simulink library "LossModelib"  (Simulink 7.8)
settings: Solver=ode45  StartTime=0.0  StopTime=10.0  RelTol=1e-3
undefined symbols (not defined in the file or in its folder): Esw_Erec, Esw_Off, Esw_On, LossSpec_Diode, LossSpec_IGBT, Page_Temp_C
libraries: simulink x12, powerlib_extras x9, fl_lib x8, powerlib x4, nesl_utility x4
settings Model: Creator=at4494  LastModifiedBy=at4494

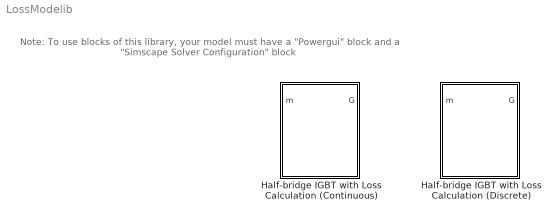
== system LossModelib ==
  note: Note: To use blocks of this library,  your model must have a "Powergui" block
      | and a "Simscape Solver Configuration" block
  Half-bridge IGBT with Loss Calculation (Continuous) : Subsystem  mask(Half-Bridge IGBT with thermal model and losses calculation){Ron=1e-3, IGBT_Type=Fuji: Half-bridge IGBT 600V/150A, PlotSpec_IGBT_On=off, ShowDataSheet_IGBT_On=off, Diode_Type=Fuji: Half-bridge IGBT 600V/150A, PlotSpec_Diode_On=off, ShowDataSheet_Diode_On=off, Tj_Init=40, PulseDuration=1e-6}
      mask prompts: Ron "Internal resistance Ron (Ohms):"; IGBT_Type "IGBT Type:"; PlotSpec_IGBT_On "Plot IGBT Characteristics"; ShowDataSheet_IGBT_On "Show Data Sheet"; Diode_Type "Diode Type:"; PlotSpec_Diode_On "Plot Diode Characteristics"; ShowDataSheet_Diode_On "Show Data Sheet"; Tj_Init "Initial Junction Temperature (degrees Celsius):"; PulseDuration "Pulse Duration for Energy-to-Power conversion (s):"
      mask init:
      | %
      | BlockName=gcb;
      | Rs=1e6;
      | Cs=inf;
      | %Tj0=273+ Tj_Init;
      | Tj0=Tj_Init;
      | %
      | load LossSpec_IGBT_Library
      | n=IGBT_Type;
      | % Add a row with 0 values for Eon and Eoff
      | E0_On=zeros(1,length(LossSpec_IGBT(n).Eon));
      | Esw_On(:,:,1)=[E0_On;LossSpec_IGBT(n).Eon(1,:)];
      | Esw_On(:,:,2)=[E0_On;LossSpec_IGBT(n).Eon(2,:)];
      | E0_Off=zeros(1,length(LossSpec_IGBT(n).Eoff));
      | Esw_Off(:,:,1)=[E0_Off;LossSpec_IGBT(n).Eoff(1,:)];
      | Esw_Off(:,:,2)=[E0_Off;LossSpec_IGBT(n).Eoff(2,:)];
      | % Create a two-element vector for Vcc (first value = 0)
      | Vcc_Esw_On=[0 LossSpec_IGBT(n).Vcc_Eon];
      | Vcc_Esw_Off=[0 LossSpec_IGBT(n).Vcc_Eoff];
      | if PlotSpec_IGBT_On==1
      |     PlotSpec1_IGBT(LossSpec_IGBT(n))
      |     set_param(BlockName,'PlotSpec_IGBT_On', 'off')
      | end
      | %
      | load LossSpec_Diode_Library
      | m=Diode_Type;
      | % Add a row with 0 values for Erec
      | E0_Erec=zeros(1,length(LossSpec_Diode(m).Erec));
      | Esw_Erec(:,:,1)=[E0_Erec;LossSpec_Diode(m).Erec(1,:)];
      | Esw_Erec(:,:,2)=[E0_Erec;LossSpec_Diode(m).Erec(2,:)];
      | % Create a two-element vector for Vcc (first value = 0)
      | Vcc_Esw_Erec=[0 LossSpec_Diode(m).Vcc_Erec];
      | if PlotSpec_Diode_On==1
      |     PlotSpec1_Diode(LossSpec_Diode(m))
      |     set_param(BlockName,'PlotSpec_Diode_On', 'off')
      | end
      | if ShowDataSheet_IGBT_On==1
      |     switch n
      |         case 1
      |     open('Spec_Fuji_IGBT600V150A.pdf')
      |         case 2
      |     open('Spec_ABB_IGBT1700V800A.pdf')
      |         case 3
      |     open('Spec_ABB_IGBT3300V250A.pdf')
      |     end
      |     set_param(BlockName,'ShowDataSheet_IGBT_On', 'off')
      | end
      | if ShowDataSheet_Diode_On==1
      |     switch m
      |         case 1
      |     open('Spec_Fuji_IGBT600V150A.pdf')
      |         case 2
      |     open('Spec_ABB_IGBT1700V800A.pdf')
      |         case 3
      |     open('Spec_ABB_IGBT3300V250A.pdf')
      |     end
      |     set_param(BlockName,'ShowDataSheet_Diode_On', 'off')
      | end
      mask StyleString: edit,popup(Fuji: Half-bridge IGBT 600V/150A|ABB: IGBT Chopper 1700V/800A|ABB: Half-Bridge IGBT 3300V/250A),checkbox,checkbox,popup(Fuji: Half-bridge IGBT 600V/150A|ABB: IGBT Chopper 1700V/800A|ABB: Half-Bridge IGBT 3300V/250A),checkbox,checkbox,edit,edit
      mask Display:
      | dX=0.02;
      | dY=0.05;
      | plot([0.19 0.292 0.292]+dX,[0.575 0.575 0.685]+dY)
      | plot([0.19 0.292 0.292]+dX,[0.195 0.195 0.305]+dY)
      | plot([0.476 0.794]+dX,[0.455 0.455]+dY)
      | plot([0.476 0.476 0.346 0.346 0.346 0.346 0.476 0.476]+dX,[0.850 0.732 0.680 0.723 0.546 0.622 0.575 0.455 ]+dY)
      | patch([0.476 0.427 0.415 0.476]+dX,[0.576 0.610 0.576 0.576]+dY)
      | %
      | plot([0.476 0.476 0.346 0.346 0.346 0.346 0.476 0.476]+dX,[0.850 0.732 0.680 0.723 0.546 0.622 0.575 0.455 ]-0.385+dY)
      | patch([0.476 0.427 0.415 0.476]+dX,[0.576 0.610 0.576 0.576]-0.385+dY)
      | %
      | plot([0.614 0.614 0.476]+dX,[0.776 0.507 0.507]+dY)
      | plot([0.614 0.476]+dX,[0.776 0.776]+dY)
      | plot([0.577 0.650]+dX,[0.679 0.679]+dY)
      | patch([0.577 0.650  0.614 0.577]+dX,[0.619 0.619 0.679 0.619]+dY)
      | %
      | plot([0.614 0.614 0.476]+dX,[0.776 0.507 0.507]-0.385+dY)
      | plot([0.614 0.476]+dX,[0.776 0.776]-0.385+dY)
      | plot([0.577 0.650]+dX,[0.679 0.679]-0.385+dY)
      | patch([0.577 0.650  0.614 0.577]+dX,[0.619 0.619 0.679 0.619]-0.385+dY)
      | %
      | port_label('RConn', 1,'+');
      | port_label('RConn', 2,'-');
      | port_label('LConn', 1,'A');
      | color('red');
      | port_label('LConn', 2,'H');
      | color('blue');
      | port_label('input', 1,'G');
  Half-bridge IGBT with Loss Calculation (Discrete) : Subsystem  mask(Half-Bridge IGBT with thermal model & losses calculation){Ron=1e-3, IGBT_Type=Fuji: Half-bridge IGBT 600V/150A, PlotSpec_IGBT_On=off, ShowDataSheet_IGBT_On=off, Diode_Type=Fuji: Half-bridge IGBT 600V/150A, PlotSpec_Diode_On=off, ShowDataSheet_Diode_On=off, Tj_Init=40, PulseDuration=1e-6, Ts=1e-6}
      mask prompts: Ron "Internal resistance Ron (Ohms):"; IGBT_Type "IGBT Type:"; PlotSpec_IGBT_On "Plot IGBT Characteristics"; ShowDataSheet_IGBT_On "Show Data Sheet"; Diode_Type "Diode Type:"; PlotSpec_Diode_On "Plot Diode Characteristics"; ShowDataSheet_Diode_On "Show Data Sheet"; Tj_Init "Initial Junction Temperature (degrees Celsius):"; PulseDuration "Pulse Duration for Energy-to-Power conversion (s):"; Ts "Sample time (s):"
      mask init:
      | %
      | BlockName=gcb;
      | Rs=1e6;
      | Cs=inf;
      | %Tj0=273+ Tj_Init;
      | Tj0=Tj_Init;
      | %
      | load LossSpec_IGBT_Library
      | n=IGBT_Type;
      | % Add a row with 0 values for Eon and Eoff
      | E0_On=zeros(1,length(LossSpec_IGBT(n).Eon));
      | Esw_On(:,:,1)=[E0_On;LossSpec_IGBT(n).Eon(1,:)];
      | Esw_On(:,:,2)=[E0_On;LossSpec_IGBT(n).Eon(2,:)];
      | E0_Off=zeros(1,length(LossSpec_IGBT(n).Eoff));
      | Esw_Off(:,:,1)=[E0_Off;LossSpec_IGBT(n).Eoff(1,:)];
      | Esw_Off(:,:,2)=[E0_Off;LossSpec_IGBT(n).Eoff(2,:)];
      | % Create a two-element vector for Vcc (first value = 0)
      | Vcc_Esw_On=[0 LossSpec_IGBT(n).Vcc_Eon];
      | Vcc_Esw_Off=[0 LossSpec_IGBT(n).Vcc_Eoff];
      | if PlotSpec_IGBT_On==1
      |     PlotSpec1_IGBT(LossSpec_IGBT(n))
      |     set_param(BlockName,'PlotSpec_IGBT_On', 'off')
      | end
      | %
      | load LossSpec_Diode_Library
      | m=Diode_Type;
      | % Add a row with 0 values for Erec
      | E0_Erec=zeros(1,length(LossSpec_Diode(m).Erec));
      | Esw_Erec(:,:,1)=[E0_Erec;LossSpec_Diode(m).Erec(1,:)];
      | Esw_Erec(:,:,2)=[E0_Erec;LossSpec_Diode(m).Erec(2,:)];
      | % Create a two-element vector for Vcc (first value = 0)
      | Vcc_Esw_Erec=[0 LossSpec_Diode(m).Vcc_Erec];
      | if PlotSpec_Diode_On==1
      |     PlotSpec1_Diode(LossSpec_Diode(m))
      |     set_param(BlockName,'PlotSpec_Diode_On', 'off')
      | end
      | if ShowDataSheet_IGBT_On==1
      |     switch n
      |         case 1
      |     open('Fuji_IGBT600V150A.pdf')
      |         case 2
      |     open('ABB_IGBT1700V800A.pdf')
      |         case 3
      |     open('ABB_IGBT3300V250A.pdf')
      |     end
      |     set_param(BlockName,'ShowDataSheet_IGBT_On', 'off')
      | end
      | if ShowDataSheet_Diode_On==1
      |     switch m
      |         case 1
      |     open('Fuji_IGBT600V150A.pdf')
      |         case 2
      |     open('ABB_IGBT1700V800A.pdf')
      |         case 3
      |     open('ABB_IGBT3300V250A.pdf')
      |     end
      |     set_param(BlockName,'ShowDataSheet_Diode_On', 'off')
      | end
      mask StyleString: edit,popup(Fuji: Half-bridge IGBT 600V/150A|ABB: IGBT Chopper 1700V/800A|ABB: Half-Bridge IGBT 3300V/250A),checkbox,checkbox,popup(Fuji: Half-bridge IGBT 600V/150A|ABB: IGBT Chopper 1700V/800A|ABB: Half-Bridge IGBT 3300V/250A),checkbox,checkbox,edit,edit,edit
      mask Display:
      | dX=0.02;
      | dY=0.05;
      | plot([0.19 0.292 0.292]+dX,[0.575 0.575 0.685]+dY)
      | plot([0.19 0.292 0.292]+dX,[0.195 0.195 0.305]+dY)
      | plot([0.476 0.794]+dX,[0.455 0.455]+dY)
      | plot([0.476 0.476 0.346 0.346 0.346 0.346 0.476 0.476]+dX,[0.850 0.732 0.680 0.723 0.546 0.622 0.575 0.455 ]+dY)
      | patch([0.476 0.427 0.415 0.476]+dX,[0.576 0.610 0.576 0.576]+dY)
      | %
      | plot([0.476 0.476 0.346 0.346 0.346 0.346 0.476 0.476]+dX,[0.850 0.732 0.680 0.723 0.546 0.622 0.575 0.455 ]-0.385+dY)
      | patch([0.476 0.427 0.415 0.476]+dX,[0.576 0.610 0.576 0.576]-0.385+dY)
      | %
      | plot([0.614 0.614 0.476]+dX,[0.776 0.507 0.507]+dY)
      | plot([0.614 0.476]+dX,[0.776 0.776]+dY)
      | plot([0.577 0.650]+dX,[0.679 0.679]+dY)
      | patch([0.577 0.650  0.614 0.577]+dX,[0.619 0.619 0.679 0.619]+dY)
      | %
      | plot([0.614 0.614 0.476]+dX,[0.776 0.507 0.507]-0.385+dY)
      | plot([0.614 0.476]+dX,[0.776 0.776]-0.385+dY)
      | plot([0.577 0.650]+dX,[0.679 0.679]-0.385+dY)
      | patch([0.577 0.650  0.614 0.577]+dX,[0.619 0.619 0.679 0.619]-0.385+dY)
      | %
      | port_label('RConn', 1,'+');
      | port_label('RConn', 2,'-');
      | port_label('LConn', 1,'A');
      | color('red');
      | port_label('LConn', 2,'H');
      | color('blue');
      | port_label('input', 1,'G');

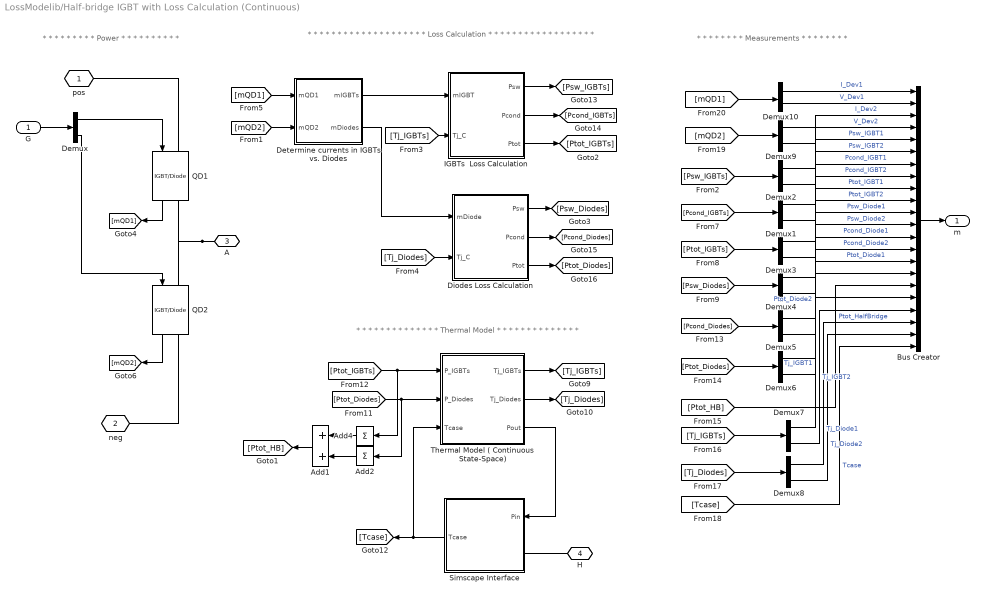
== system LossModelib/Half-bridge IGBT with Loss Calculation (Continuous) ==
  note: * * * * * * * * * Power * * * * * * * * * *
  note: * * * * * * * * * * * * * * * * * * * * Loss Calculation * * * * * * * * * * * * * * * * * *
  note: * * * * * * * * * * * * * * Thermal Model * * * * * * * * * * * * * *
  note: * * * * * * * * Measurements * * * * * * * *
  G : Inport  PortDimensions=2
  Add1 : Sum
  Add2 : Sum  Inputs=+
  Add4 : Sum  Inputs=+
  Bus Creator : BusCreator  Inputs=22
  Demux{,1..10} (11 alike) : Demux  Outputs=2
  Determine currents in IGBTs vs. Diodes : Subsystem
  Diodes Loss Calculation : Subsystem
  IGBTs  Loss Calculation : Subsystem
  QD1 : powerlib/Power Electronics/IGBT//Diode  Ron=Ron  Rs=Rs  Cs=Cs  Measurements=on
  QD2 : powerlib/Power Electronics/IGBT//Diode  Ron=Ron  Rs=Rs  Cs=Cs  Measurements=on
  Simscape Interface : Subsystem
  Thermal Model ( Continuous State-Space) : Subsystem  mask(State-Space Thermal Model (Junction-to-Case)){Zth_IGBT=[ LossSpec_IGBT(n).Rth_jc    LossSpec_IGBT(n).Cth_j ], Zth_Diode=[ LossSpec_Diode(m).Rth_jc    LossSpec_Diode(m).Cth_j ], Tj0=Tj0}
      mask prompts: Zth_IGBT "IGBT Thermal Impedance [ Rth (K/W)  Cth (J/K) ]:"; Zth_Diode "Diode Thermal Impedance [ Rth (K/W)  Cth (J/K) ]:"; Tj0 "Junction Initial Temperature (C)"
      mask init:
      | %
      | Rth_IGBT= Zth_IGBT(1);
      | Cth_IGBT= Zth_IGBT(2);
      | Rth_Diode= Zth_Diode(1);
      | Cth_Diode= Zth_Diode(2);
      | %
      | Ac_IGBT= -1/(Rth_IGBT*Cth_IGBT);
      | Bc_IGBT= [ 1/(Rth_IGBT*Cth_IGBT)  1/Cth_IGBT ];
      | Cc_IGBT= [ 1; 1/Rth_IGBT ];
      | Dc_IGBT= [ 0  0; -1/Rth_IGBT 0 ];
      | %
      | Ac_Diode= -1/(Rth_Diode*Cth_Diode);
      | Bc_Diode= [ 1/(Rth_Diode*Cth_Diode)  1/Cth_Diode ];
      | Cc_Diode= [ 1; 1/Rth_Diode ];
      | Dc_Diode= [ 0  0; -1/Rth_Diode 0 ];
      | %
      | x0c=Tj0;
      | %
  pos : PMIOPort  Port=1  Side=Right
  neg : PMIOPort  Port=2  Side=Right
  A : PMIOPort  Port=3  Side=Left
  H : PMIOPort  Port=4  Side=Left
  m : Outport
  wires:
  Simscape Interface/1(Tcase) -> Thermal Model ( Continuous State-Space)/3(Tcase), [Tcase]
  Thermal Model ( Continuous State-Space)/3(Pout) -> Simscape Interface/1(Pin)
  [Ptot_IGBTs] -> Thermal Model ( Continuous State-Space)/1(P_IGBTs), Add4/1
  [Ptot_Diodes] -> Thermal Model ( Continuous State-Space)/2(P_Diodes), Add2/1
  Thermal Model ( Continuous State-Space)/1(Tj_IGBTs) -> [Tj_IGBTs]
  Thermal Model ( Continuous State-Space)/2(Tj_Diodes) -> [Tj_Diodes]
  QD1/1 -> [mQD1]
  QD2/1 -> [mQD2]
  Demux/1 -> QD1/1
  G/1 -> Demux/1
  Demux/2 -> QD2/1
  IGBTs  Loss Calculation/2(Pcond) -> [Pcond_IGBTs]
  [mQD1] -> Determine currents in IGBTs vs. Diodes/1(mQD1)
  [mQD2] -> Determine currents in IGBTs vs. Diodes/2(mQD2)
  Determine currents in IGBTs vs. Diodes/1(mIGBTs) -> IGBTs  Loss Calculation/1(mIGBT)
  Determine currents in IGBTs vs. Diodes/2(mDiodes) -> Diodes Loss Calculation/1(mDiode)
  IGBTs  Loss Calculation/1(Psw) -> [Psw_IGBTs]
  [Tj_IGBTs] -> IGBTs  Loss Calculation/2(Tj_C)
  [Tj_Diodes] -> Diodes Loss Calculation/2(Tj_C)
  IGBTs  Loss Calculation/3(Ptot) -> [Ptot_IGBTs]
  Diodes Loss Calculation/1(Psw) -> [Psw_Diodes]
  Diodes Loss Calculation/2(Pcond) -> [Pcond_Diodes]
  Diodes Loss Calculation/3(Ptot) -> [Ptot_Diodes]
  Bus Creator/1 -> m/1
  [Psw_IGBTs] -> Demux2/1
  [Pcond_IGBTs] -> Demux1/1
  [Ptot_IGBTs] -> Demux3/1
  [Psw_Diodes] -> Demux4/1
  [Pcond_Diodes] -> Demux5/1
  [Ptot_Diodes] -> Demux6/1
  Add1/1 -> [Ptot_HB]
  [Tj_IGBTs] -> Demux7/1
  [Tj_Diodes] -> Demux8/1
  [mQD1] -> Demux10/1
  [mQD2] -> Demux9/1
  Demux10/1 -> Bus Creator/1  "I_Dev1"
  Demux10/2 -> Bus Creator/2  "V_Dev1"
  Demux9/1 -> Bus Creator/3  "I_Dev2"
  Demux9/2 -> Bus Creator/4  "V_Dev2"
  Demux2/1 -> Bus Creator/5  "Psw_IGBT1"
  Demux2/2 -> Bus Creator/6  "Psw_IGBT2"
  Demux1/1 -> Bus Creator/7  "Pcond_IGBT1"
  Demux1/2 -> Bus Creator/8  "Pcond_IGBT2"
  Demux3/1 -> Bus Creator/9  "Ptot_IGBT1"
  Demux3/2 -> Bus Creator/10  "Ptot_IGBT2"
  Demux4/1 -> Bus Creator/11  "Psw_Diode1"
  Demux4/2 -> Bus Creator/12  "Psw_Diode2"
  Demux5/1 -> Bus Creator/13  "Pcond_Diode1"
  Demux5/2 -> Bus Creator/14  "Pcond_Diode2"
  Demux6/1 -> Bus Creator/15  "Ptot_Diode1"
  Demux6/2 -> Bus Creator/16  "Ptot_Diode2"
  [Ptot_HB] -> Bus Creator/17  "Ptot_HalfBridge"
  Demux7/1 -> Bus Creator/18  "Tj_IGBT1"
  Demux7/2 -> Bus Creator/19  "Tj_IGBT2"
  Demux8/1 -> Bus Creator/20  "Tj_Diode1"
  Demux8/2 -> Bus Creator/21  "Tj_Diode2"
  [Tcase] -> Bus Creator/22  "Tcase"
  Add4/1 -> Add1/1
  Add2/1 -> Add1/2
  connections:
  H/RConn1 -- Simscape Interface/LConn1
  A/RConn1 -- QD2/LConn1 -- QD1/RConn1
  pos/RConn1 -- QD1/LConn1
  neg/RConn1 -- QD2/RConn1

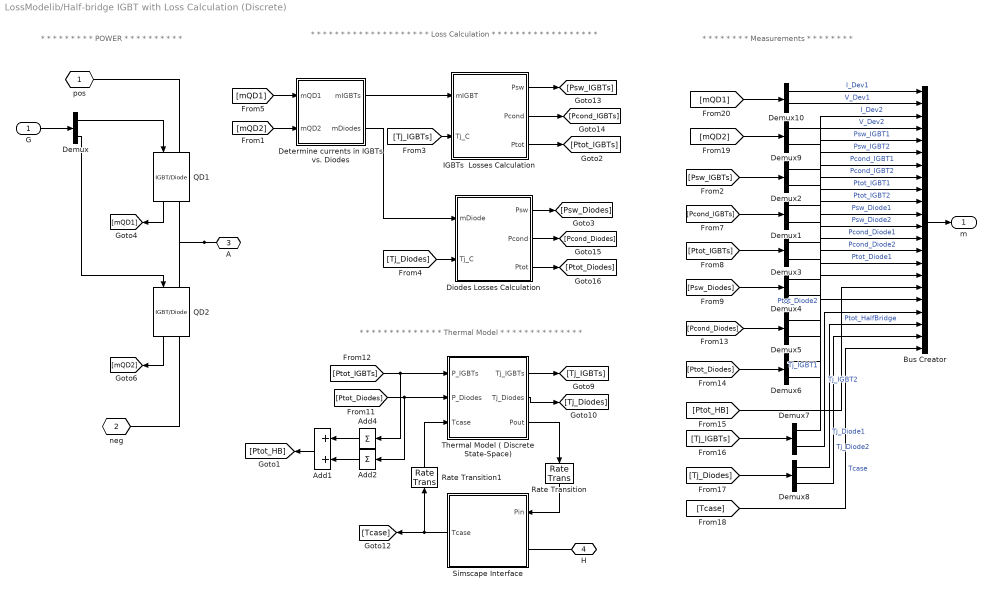
== system LossModelib/Half-bridge IGBT with Loss Calculation (Discrete) ==
  note: * * * * * * * * * POWER * * * * * * * * * *
  note: * * * * * * * * * * * * * * * * * * * * Loss Calculation * * * * * * * * * * * * * * * * * *
  note: * * * * * * * * * * * * * * Thermal Model * * * * * * * * * * * * * *
  note: * * * * * * * * Measurements * * * * * * * *
  G : Inport  PortDimensions=2
  Add1 : Sum
  Add2 : Sum  Inputs=+
  Add4 : Sum  Inputs=+
  Bus Creator : BusCreator  Inputs=22
  Demux{,1..10} (11 alike) : Demux  Outputs=2
  Determine currents in IGBTs vs. Diodes : Subsystem
  Diodes Losses Calculation : Subsystem
  IGBTs  Losses Calculation : Subsystem
  QD1 : powerlib/Power Electronics/IGBT//Diode  Ron=Ron  Rs=Rs  Cs=Cs  Measurements=on
  QD2 : powerlib/Power Electronics/IGBT//Diode  Ron=Ron  Rs=Rs  Cs=Cs  Measurements=on
  Rate Transition : RateTransition  OutPortSampleTime=100e-6
  Rate Transition1 : RateTransition  OutPortSampleTime=Ts
  Simscape Interface : Subsystem
  Thermal Model ( Discrete State-Space) : Subsystem  mask(State-Space Thermal Model (Junction-to-Case)){Zth_IGBT=[ LossSpec_IGBT(n).Rth_jc    LossSpec_IGBT(n).Cth_j ], Zth_Diode=[ LossSpec_Diode(m).Rth_jc    LossSpec_Diode(m).Cth_j], Tj0=Tj0, Ts=Ts}
      mask prompts: Zth_IGBT "IGBT Thermal Impedance [ Rth (K/W)  Cth (J/K) ]:"; Zth_Diode "Diode Thermal Impedance [ Rth (K/W)  Cth (J/K) ]:"; Tj0 "Junction Initial Temperature (C)"; Ts "Sample time (s):"
      mask init:
      | %
      | Rth_IGBT= Zth_IGBT(1);
      | Cth_IGBT= Zth_IGBT(2);
      | Rth_Diode= Zth_Diode(1);
      | Cth_Diode= Zth_Diode(2);
      | %
      | Ac_IGBT= -1/(Rth_IGBT*Cth_IGBT);
      | Bc_IGBT= [ 1/(Rth_IGBT*Cth_IGBT)  1/Cth_IGBT ];
      | Cc_IGBT= [ 1; 1/Rth_IGBT ];
      | Dc_IGBT= [ 0  0; -1/Rth_IGBT 0 ];
      | %
      | Ac_Diode= -1/(Rth_Diode*Cth_Diode);
      | Bc_Diode= [ 1/(Rth_Diode*Cth_Diode)  1/Cth_Diode ];
      | Cc_Diode= [ 1; 1/Rth_Diode ];
      | Dc_Diode= [ 0  0; -1/Rth_Diode 0 ];
      | %
      | x0c=Tj0;
      | %
      | %  Conversion to discrete transfer function
      | nstates = size(Ac_IGBT,1);
      | invexp = inv(eye(nstates) - (Ts/2)*Ac_IGBT);
      | Ad_IGBT = invexp*(eye(nstates) + (Ts/2)*Ac_IGBT);
      | Bd_IGBT = invexp*Bc_IGBT;
      | Cd_IGBT = Cc_IGBT*invexp*Ts;
      | Dd_IGBT = Cc_IGBT*invexp*Bc_IGBT*(Ts/2) + Dc_IGBT;
      | %
      | x0c=Tj0;
      | I=eye(size(Ac_IGBT));
      | x0d=(I-Ac_IGBT*Ts/2)*x0c/Ts;
      | %
      | %  Conversion to discrete transfer function
      | nstates = size(Ac_Diode,1);
      | invexp = inv(eye(nstates) - (Ts/2)*Ac_Diode);
      | Ad_Diode = invexp*(eye(nstates) + (Ts/2)*Ac_Diode);
      | Bd_Diode = invexp*Bc_Diode;
      | Cd_Diode = Cc_Diode*invexp*Ts;
      | Dd_Diode = Cc_Diode*invexp*Bc_Diode*(Ts/2) + Dc_Diode;
      | %
  pos : PMIOPort  Port=1  Side=Right
  neg : PMIOPort  Port=2  Side=Right
  A : PMIOPort  Port=3  Side=Left
  H : PMIOPort  Port=4  Side=Left
  m : Outport
  wires:
  Simscape Interface/1(Tcase) -> [Tcase], Rate Transition1/1
  Thermal Model ( Discrete State-Space)/3(Pout) -> Rate Transition/1
  [Ptot_IGBTs] -> Add4/1, Thermal Model ( Discrete State-Space)/1(P_IGBTs)
  [Ptot_Diodes] -> Add2/1, Thermal Model ( Discrete State-Space)/2(P_Diodes)
  Thermal Model ( Discrete State-Space)/1(Tj_IGBTs) -> [Tj_IGBTs]
  Thermal Model ( Discrete State-Space)/2(Tj_Diodes) -> [Tj_Diodes]
  QD1/1 -> [mQD1]
  QD2/1 -> [mQD2]
  Demux/1 -> QD1/1
  G/1 -> Demux/1
  Demux/2 -> QD2/1
  IGBTs  Losses Calculation/2(Pcond) -> [Pcond_IGBTs]
  [mQD1] -> Determine currents in IGBTs vs. Diodes/1(mQD1)
  [mQD2] -> Determine currents in IGBTs vs. Diodes/2(mQD2)
  Determine currents in IGBTs vs. Diodes/1(mIGBTs) -> IGBTs  Losses Calculation/1(mIGBT)
  Determine currents in IGBTs vs. Diodes/2(mDiodes) -> Diodes Losses Calculation/1(mDiode)
  IGBTs  Losses Calculation/1(Psw) -> [Psw_IGBTs]
  [Tj_IGBTs] -> IGBTs  Losses Calculation/2(Tj_C)
  [Tj_Diodes] -> Diodes Losses Calculation/2(Tj_C)
  IGBTs  Losses Calculation/3(Ptot) -> [Ptot_IGBTs]
  Diodes Losses Calculation/1(Psw) -> [Psw_Diodes]
  Diodes Losses Calculation/2(Pcond) -> [Pcond_Diodes]
  Diodes Losses Calculation/3(Ptot) -> [Ptot_Diodes]
  Bus Creator/1 -> m/1
  [Psw_IGBTs] -> Demux2/1
  [Pcond_IGBTs] -> Demux1/1
  [Ptot_IGBTs] -> Demux3/1
  [Psw_Diodes] -> Demux4/1
  [Pcond_Diodes] -> Demux5/1
  [Ptot_Diodes] -> Demux6/1
  Add1/1 -> [Ptot_HB]
  [Tj_IGBTs] -> Demux7/1
  [Tj_Diodes] -> Demux8/1
  [mQD1] -> Demux10/1
  [mQD2] -> Demux9/1
  Demux10/1 -> Bus Creator/1  "I_Dev1"
  Demux10/2 -> Bus Creator/2  "V_Dev1"
  Demux9/1 -> Bus Creator/3  "I_Dev2"
  Demux9/2 -> Bus Creator/4  "V_Dev2"
  Demux2/1 -> Bus Creator/5  "Psw_IGBT1"
  Demux2/2 -> Bus Creator/6  "Psw_IGBT2"
  Demux1/1 -> Bus Creator/7  "Pcond_IGBT1"
  Demux1/2 -> Bus Creator/8  "Pcond_IGBT2"
  Demux3/1 -> Bus Creator/9  "Ptot_IGBT1"
  Demux3/2 -> Bus Creator/10  "Ptot_IGBT2"
  Demux4/1 -> Bus Creator/11  "Psw_Diode1"
  Demux4/2 -> Bus Creator/12  "Psw_Diode2"
  Demux5/1 -> Bus Creator/13  "Pcond_Diode1"
  Demux5/2 -> Bus Creator/14  "Pcond_Diode2"
  Demux6/1 -> Bus Creator/15  "Ptot_Diode1"
  Demux6/2 -> Bus Creator/16  "Ptot_Diode2"
  [Ptot_HB] -> Bus Creator/17  "Ptot_HalfBridge"
  Demux7/1 -> Bus Creator/18  "Tj_IGBT1"
  Demux7/2 -> Bus Creator/19  "Tj_IGBT2"
  Demux8/1 -> Bus Creator/20  "Tj_Diode1"
  Demux8/2 -> Bus Creator/21  "Tj_Diode2"
  [Tcase] -> Bus Creator/22  "Tcase"
  Add4/1 -> Add1/1
  Add2/1 -> Add1/2
  Rate Transition1/1 -> Thermal Model ( Discrete State-Space)/3(Tcase)
  Rate Transition/1 -> Simscape Interface/1(Pin)
  connections:
  H/RConn1 -- Simscape Interface/LConn1
  A/RConn1 -- QD2/LConn1 -- QD1/RConn1
  pos/RConn1 -- QD1/LConn1
  neg/RConn1 -- QD2/RConn1

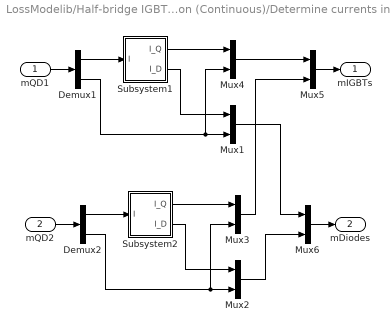
== system LossModelib/Half-bridge IGBT with Loss Calculation (Continuous)/Determine currents in IGBTs vs. Diodes ==
  mQD1 : Inport
  mQD2 : Inport  Port=2
  Demux1 : Demux  Outputs=2
  Demux2 : Demux  Outputs=2
  Mux{1..6} (6 alike) : Mux  Inputs=2
  Subsystem1 : Subsystem
  Subsystem2 : Subsystem
  mIGBTs : Outport
  mDiodes : Outport  Port=2
  wires:
  Demux1/1 -> Subsystem1/1(I)
  Subsystem1/1(I_Q) -> Mux4/1
  Demux1/2 -> Mux1/2, Mux4/2
  Subsystem1/2(I_D) -> Mux1/1
  Demux2/1 -> Subsystem2/1(I)
  Subsystem2/1(I_Q) -> Mux3/1
  Demux2/2 -> Mux3/2, Mux2/2
  Subsystem2/2(I_D) -> Mux2/1
  Mux4/1 -> Mux5/1
  Mux3/1 -> Mux5/2
  Mux1/1 -> Mux6/1
  Mux2/1 -> Mux6/2
  mQD1/1 -> Demux1/1
  Mux5/1 -> mIGBTs/1
  mQD2/1 -> Demux2/1
  Mux6/1 -> mDiodes/1

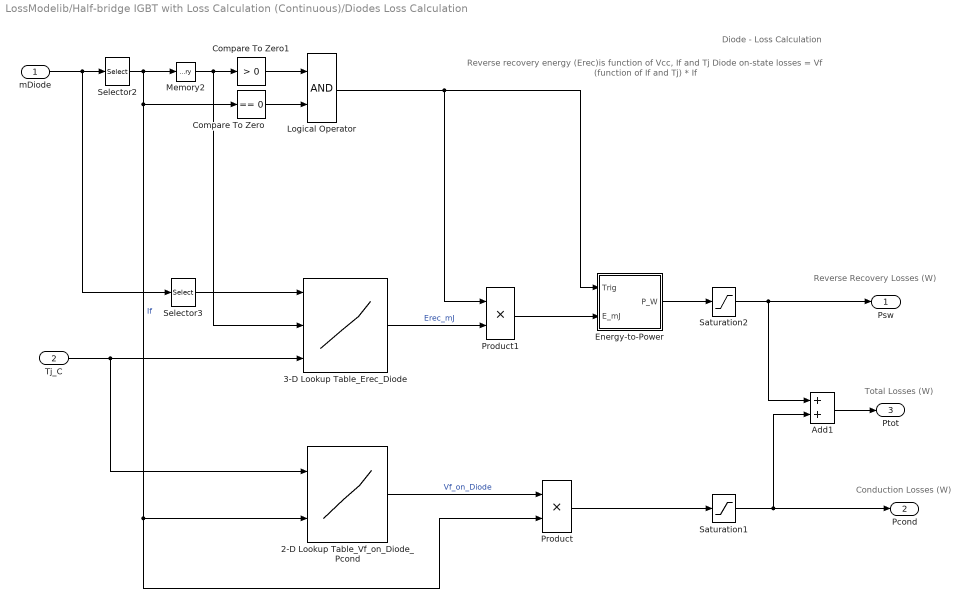
== system LossModelib/Half-bridge IGBT with Loss Calculation (Continuous)/Diodes Loss Calculation ==
  note: Conduction Losses (W)
  note: Total Losses (W)
  note: Reverse Recovery Losses (W)
  note: Reverse recovery energy (Erec)is function of Vcc, If and Tj
      | Diode on-state losses = Vf (function of If and Tj) * If
  note: Diode - Loss Calculation
  mDiode : Inport  PortDimensions=4
  Tj_C : Inport  Port=2
  2-D Lookup Table_Vf_on_Diode_Pcond : Lookup_n-D  BreakpointsForDimension1=LossSpec_Diode(m).Tj_OnState  BreakpointsForDimension2=LossSpec_Diode(m).If_OnState  BreakpointsForDimension3=Page_Temp_C  Table=LossSpec_Diode(m).Vf_OnState  RndMeth=Simplest  InputSameDT=on
  3-D Lookup Table_Erec_Diode : Lookup_n-D  NumberOfTableDimensions=3  BreakpointsForDimension1=Vcc_Esw_Erec  BreakpointsForDimension2=LossSpec_Diode(m).If_Erec  BreakpointsForDimension3=LossSpec_Diode(m).Tj_Erec  Table=Esw_Erec  RndMeth=Simplest  InputSameDT=on
  Add1 : Sum
  Compare To Zero : simulink/Logic and Bit Operations/Compare To Zero  relop===  OutDataTypeStr=boolean
  Compare To Zero1 : simulink/Logic and Bit Operations/Compare To Zero  relop=>  OutDataTypeStr=boolean
  "Energy-to-Power " : Subsystem  mask{PulseDuration=PulseDuration}
      mask prompts: PulseDuration "Pulse Duration (s):"
  Logical Operator : Logic  AllPortsSameDT=off  OutDataTypeStr=float('double')
  Memory2 : Memory
  Product : Product  RndMeth=Zero
  Product1 : Product  RndMeth=Zero
  Saturation1 : Saturate  UpperLimit=inf  LowerLimit=0
  Saturation2 : Saturate  UpperLimit=inf  LowerLimit=0
  Selector2 : Selector  InputPortWidth=4  IndexOptions=Index vector (dialog)  Indices="[ 1  3 ]"  OutputSizes=1
  Selector3 : Selector  InputPortWidth=4  IndexOptions=Index vector (dialog)  Indices=[ 2 4 ]  OutputSizes=1
  Psw : Outport
  Pcond : Outport  Port=2
  Ptot : Outport  Port=3
  wires:
  "Energy-to-Power "/1(P_W) -> Saturation2/1
  Product1/1 -> "Energy-to-Power "/2(E_mJ)
  Product/1 -> Saturation1/1
  Tj_C/1 -> 2-D Lookup Table_Vf_on_Diode_Pcond/1, 3-D Lookup Table_Erec_Diode/3
  2-D Lookup Table_Vf_on_Diode_Pcond/1 -> Product/1  "Vf_on_Diode"
  Add1/1 -> Ptot/1
  Compare To Zero1/1 -> Logical Operator/1
  Compare To Zero/1 -> Logical Operator/2
  Logical Operator/1 -> "Energy-to-Power "/1(Trig), Product1/1
  3-D Lookup Table_Erec_Diode/1 -> Product1/2  "Erec_mJ"
  Selector2/1 -> Memory2/1, Compare To Zero/1, 2-D Lookup Table_Vf_on_Diode_Pcond/2, Product/2  "If"
  mDiode/1 -> Selector2/1, Selector3/1
  Selector3/1 -> 3-D Lookup Table_Erec_Diode/1
  Memory2/1 -> Compare To Zero1/1, 3-D Lookup Table_Erec_Diode/2
  Saturation2/1 -> Psw/1, Add1/1
  Saturation1/1 -> Pcond/1, Add1/2

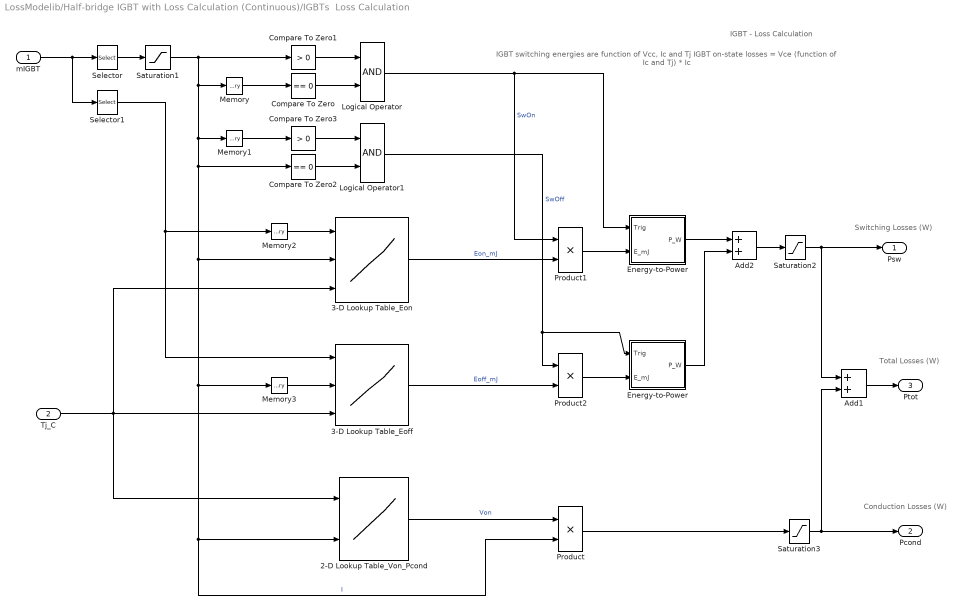
== system LossModelib/Half-bridge IGBT with Loss Calculation (Continuous)/IGBTs  Loss Calculation ==
  note: IGBT switching energies are function of Vcc, Ic and Tj
      | IGBT on-state losses = Vce (function of Ic and Tj) * Ic
  note: Total Losses (W)
  note: Conduction Losses (W)
  note: Switching Losses (W)
  note: IGBT - Loss Calculation
  mIGBT : Inport  PortDimensions=4
  Tj_C : Inport  Port=2
  2-D Lookup Table_Von_Pcond : Lookup_n-D  BreakpointsForDimension1=LossSpec_IGBT(n).Tj_OnState  BreakpointsForDimension2=LossSpec_IGBT(n).Ic_OnState  BreakpointsForDimension3=Page_Temp_C  Table=LossSpec_IGBT(n).Vce_OnState  RndMeth=Simplest  InputSameDT=on
  3-D Lookup Table_Eoff : Lookup_n-D  NumberOfTableDimensions=3  BreakpointsForDimension1=Vcc_Esw_Off  BreakpointsForDimension2=LossSpec_IGBT(n).Ic_Eoff  BreakpointsForDimension3=LossSpec_IGBT(n).Tj_Eoff  Table=Esw_Off  RndMeth=Simplest  InputSameDT=on
  3-D Lookup Table_Eon : Lookup_n-D  NumberOfTableDimensions=3  BreakpointsForDimension1=Vcc_Esw_On  BreakpointsForDimension2=LossSpec_IGBT(n).Ic_Eon  BreakpointsForDimension3=LossSpec_IGBT(n).Tj_Eon  Table=Esw_On  RndMeth=Simplest  InputSameDT=on
  Add1 : Sum
  Add2 : Sum
  Compare To Zero : simulink/Logic and Bit Operations/Compare To Zero  relop===  OutDataTypeStr=boolean
  Compare To Zero1 : simulink/Logic and Bit Operations/Compare To Zero  relop=>  OutDataTypeStr=boolean
  Compare To Zero2 : simulink/Logic and Bit Operations/Compare To Zero  relop===  OutDataTypeStr=boolean
  Compare To Zero3 : simulink/Logic and Bit Operations/Compare To Zero  relop=>  OutDataTypeStr=boolean
  Energy-to-Power : Subsystem  mask{PulseDuration=PulseDuration}
      mask prompts: PulseDuration "Pulse Duration (s):"
  "Energy-to-Power " : Subsystem  mask{PulseDuration=PulseDuration}
      mask prompts: PulseDuration "Pulse Duration (s):"
  Logical Operator : Logic  AllPortsSameDT=off  OutDataTypeStr=float('double')
  Logical Operator1 : Logic  AllPortsSameDT=off  OutDataTypeStr=float('double')
  Memory{,1..3} (4 alike) : Memory
  Product : Product  RndMeth=Zero
  Product1 : Product  RndMeth=Zero
  Product2 : Product  RndMeth=Zero
  Saturation1 : Saturate  UpperLimit=inf  LowerLimit=0
  Saturation2 : Saturate  UpperLimit=inf  LowerLimit=0
  Saturation3 : Saturate  UpperLimit=inf  LowerLimit=0
  Selector : Selector  InputPortWidth=4  IndexOptions=Index vector (dialog)  Indices="[ 1  3 ]"  OutputSizes=1
  Selector1 : Selector  InputPortWidth=4  IndexOptions=Index vector (dialog)  Indices=[ 2 4 ]  OutputSizes=1
  Psw : Outport
  Pcond : Outport  Port=2
  Ptot : Outport  Port=3
  wires:
  Energy-to-Power/1(P_W) -> Add2/2
  Product2/1 -> Energy-to-Power/2(E_mJ)
  Product1/1 -> "Energy-to-Power "/2(E_mJ)
  "Energy-to-Power "/1(P_W) -> Add2/1
  2-D Lookup Table_Von_Pcond/1 -> Product/1  "Von"
  Tj_C/1 -> 3-D Lookup Table_Eoff/3, 2-D Lookup Table_Von_Pcond/1, 3-D Lookup Table_Eon/3
  Product/1 -> Saturation3/1
  3-D Lookup Table_Eoff/1 -> Product2/2  "Eoff_mJ"
  3-D Lookup Table_Eon/1 -> Product1/2  "Eon_mJ"
  Memory3/1 -> 3-D Lookup Table_Eoff/2
  Memory2/1 -> 3-D Lookup Table_Eon/1
  Selector/1 -> Saturation1/1
  Add1/1 -> Ptot/1
  mIGBT/1 -> Selector/1, Selector1/1
  Memory/1 -> Compare To Zero/1
  Saturation1/1 -> Compare To Zero1/1, Memory/1, Memory1/1, 3-D Lookup Table_Eon/2, Memory3/1, 2-D Lookup Table_Von_Pcond/2, Product/2, Compare To Zero2/1  "I"
  Compare To Zero1/1 -> Logical Operator/1
  Compare To Zero/1 -> Logical Operator/2
  Logical Operator/1 -> "Energy-to-Power "/1(Trig), Product1/1  "SwOn"
  Selector1/1 -> Memory2/1, 3-D Lookup Table_Eoff/1
  Compare To Zero3/1 -> Logical Operator1/1
  Compare To Zero2/1 -> Logical Operator1/2
  Logical Operator1/1 -> Energy-to-Power/1(Trig), Product2/1  "SwOff"
  Memory1/1 -> Compare To Zero3/1
  Add2/1 -> Saturation2/1
  Saturation2/1 -> Psw/1, Add1/1
  Saturation3/1 -> Pcond/1, Add1/2

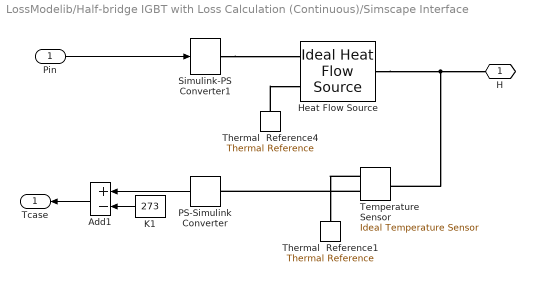
== system LossModelib/Half-bridge IGBT with Loss Calculation (Continuous)/Simscape Interface ==
  Pin : Inport
  Add1 : Sum  Inputs=+-
  Heat Flow Source : fl_lib/Thermal/Thermal Sources/Ideal Heat Flow Source  Q_Log=off  T_Log=off  LocalVarNames=|Q|T  LocalVarDescs=|Q|T  LocalVarLogging=[0 0]
  K1 : Constant  Value=273
  PS-Simulink Converter : nesl_utility/PS-Simulink Converter  PhysicalDomain=network_engine_domain  LeftPortType=input  RightPortType=output  SubClassName=ps_output  Unit=1  AffineConversion=off
  Simulink-PS Converter1 : nesl_utility/Simulink-PS Converter  PhysicalDomain=network_engine_domain  LeftPortType=input  RightPortType=output  SubClassName=ps_input  Unit=1  AffineConversion=off  InputFilterTimeConstant=1e-4  UdotUserProvided=0
  Temperature Sensor : fl_lib/Thermal/Thermal Sensors/Ideal Temperature Sensor  Qs_Log=off  Ts_Log=off  LocalVarNames=|Qs|Ts  LocalVarDescs=|Qs|Ts  LocalVarLogging=[0 0]
  Thermal  Reference1 : fl_lib/Thermal/Thermal Elements/Thermal Reference  Q_Log=off  LocalVarNames=|Q  LocalVarDescs=|Q  LocalVarLogging=0
  Thermal  Reference4 : fl_lib/Thermal/Thermal Elements/Thermal Reference  Q_Log=off  LocalVarNames=|Q  LocalVarDescs=|Q  LocalVarLogging=0
  H : PMIOPort  Port=1  Side=Left
  Tcase : Outport
  wires:
  Add1/1 -> Tcase/1
  PS-Simulink Converter/1 -> Add1/1
  K1/1 -> Add1/2
  Pin/1 -> Simulink-PS Converter1/1
  connections:
  Thermal  Reference4/LConn1 -- Heat Flow Source/RConn2
  Temperature Sensor/RConn1 -- Thermal  Reference1/LConn1
  Temperature Sensor/RConn2 -- PS-Simulink Converter/LConn1
  Simulink-PS Converter1/RConn1 -- Heat Flow Source/RConn1
  Temperature Sensor/LConn1 -- H/RConn1 -- Heat Flow Source/LConn1

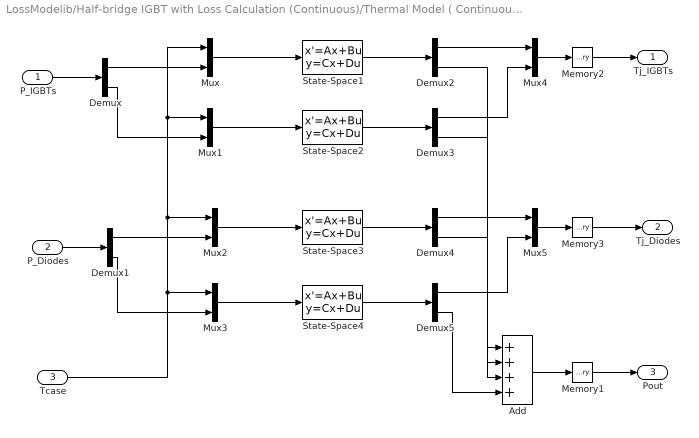
== system LossModelib/Half-bridge IGBT with Loss Calculation (Continuous)/Thermal Model ( Continuous State-Space) ==
  P_IGBTs : Inport  PortDimensions=2
  P_Diodes : Inport  Port=2  PortDimensions=2
  Tcase : Inport  Port=3  PortDimensions=1
  Add : Sum  Inputs=++++
  Demux{,1..5} (6 alike) : Demux  Outputs=2
  Memory1 : Memory
  Memory2 : Memory  X0=x0c
  Memory3 : Memory  X0=x0c
  Mux{,1..5} (6 alike) : Mux  Inputs=2
  State-Space1 : StateSpace  A=Ac_IGBT  B=Bc_IGBT  C=Cc_IGBT  D=Dc_IGBT  X0=x0c
  State-Space2 : StateSpace  A=Ac_IGBT  B=Bc_IGBT  C=Cc_IGBT  D=Dc_IGBT  X0=x0c
  State-Space3 : StateSpace  A=Ac_Diode  B=Bc_Diode  C=Cc_Diode  D=Dc_Diode  X0=x0c
  State-Space4 : StateSpace  A=Ac_Diode  B=Bc_Diode  C=Cc_Diode  D=Dc_Diode  X0=x0c
  Tj_IGBTs : Outport
  Tj_Diodes : Outport  Port=2
  Pout : Outport  Port=3
  wires:
  State-Space3/1 -> Demux4/1
  State-Space2/1 -> Demux3/1
  State-Space4/1 -> Demux5/1
  State-Space1/1 -> Demux2/1
  Mux3/1 -> State-Space4/1
  Mux2/1 -> State-Space3/1
  Mux1/1 -> State-Space2/1
  Mux/1 -> State-Space1/1
  Add/1 -> Memory1/1
  Demux1/1 -> Mux2/2
  Demux/1 -> Mux/2
  Demux/2 -> Mux1/2
  Demux1/2 -> Mux3/2
  Demux2/1 -> Mux4/1
  Demux3/1 -> Mux4/2
  Mux4/1 -> Memory2/1
  Demux4/1 -> Mux5/1
  Demux5/1 -> Mux5/2
  Demux2/2 -> Add/1
  Demux3/2 -> Add/2
  Demux4/2 -> Add/3
  Demux5/2 -> Add/4
  Mux5/1 -> Memory3/1
  P_IGBTs/1 -> Demux/1
  P_Diodes/1 -> Demux1/1
  Tcase/1 -> Mux3/1, Mux/1, Mux1/1, Mux2/1
  Memory1/1 -> Pout/1
  Memory3/1 -> Tj_Diodes/1
  Memory2/1 -> Tj_IGBTs/1

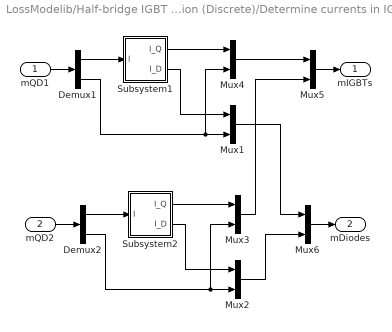
== system LossModelib/Half-bridge IGBT with Loss Calculation (Discrete)/Determine currents in IGBTs vs. Diodes ==
  mQD1 : Inport
  mQD2 : Inport  Port=2
  Demux1 : Demux  Outputs=2
  Demux2 : Demux  Outputs=2
  Mux{1..6} (6 alike) : Mux  Inputs=2
  Subsystem1 : Subsystem
  Subsystem2 : Subsystem
  mIGBTs : Outport
  mDiodes : Outport  Port=2
  wires:
  Demux1/1 -> Subsystem1/1(I)
  Subsystem1/1(I_Q) -> Mux4/1
  Demux1/2 -> Mux1/2, Mux4/2
  Subsystem1/2(I_D) -> Mux1/1
  Demux2/1 -> Subsystem2/1(I)
  Subsystem2/1(I_Q) -> Mux3/1
  Demux2/2 -> Mux3/2, Mux2/2
  Subsystem2/2(I_D) -> Mux2/1
  Mux4/1 -> Mux5/1
  Mux3/1 -> Mux5/2
  Mux1/1 -> Mux6/1
  Mux2/1 -> Mux6/2
  mQD1/1 -> Demux1/1
  Mux5/1 -> mIGBTs/1
  mQD2/1 -> Demux2/1
  Mux6/1 -> mDiodes/1

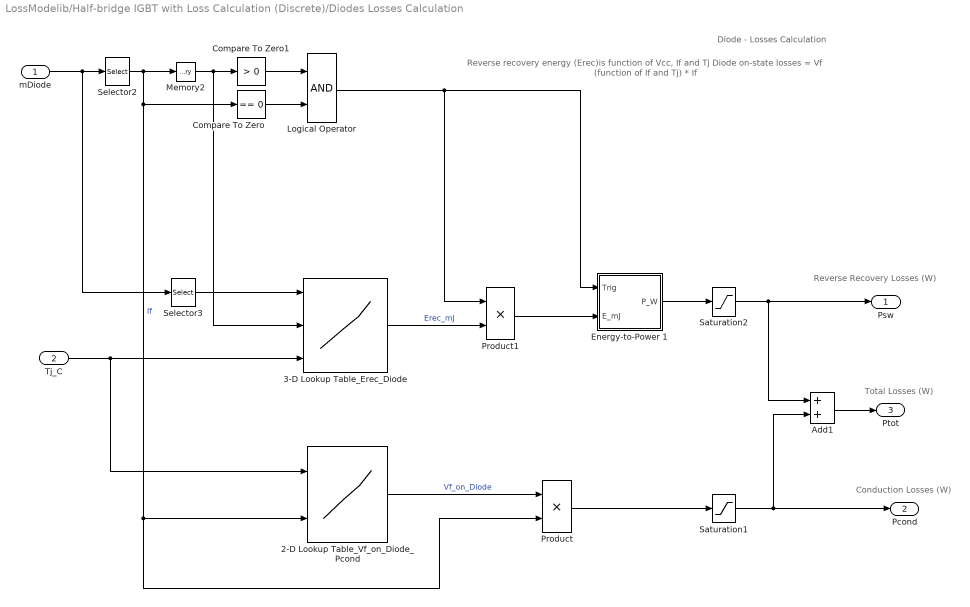
== system LossModelib/Half-bridge IGBT with Loss Calculation (Discrete)/Diodes Losses Calculation ==
  note: Conduction Losses (W)
  note: Total Losses (W)
  note: Reverse Recovery Losses (W)
  note: Reverse recovery energy (Erec)is function of Vcc, If and Tj
      | Diode on-state losses = Vf (function of If and Tj) * If
  note: Diode - Losses Calculation
  mDiode : Inport  PortDimensions=4
  Tj_C : Inport  Port=2
  2-D Lookup Table_Vf_on_Diode_Pcond : Lookup_n-D  BreakpointsForDimension1=LossSpec_Diode(m).Tj_OnState  BreakpointsForDimension2=LossSpec_Diode(m).If_OnState  BreakpointsForDimension3=Page_Temp_C  Table=LossSpec_Diode(m).Vf_OnState  RndMeth=Simplest  InputSameDT=on
  3-D Lookup Table_Erec_Diode : Lookup_n-D  NumberOfTableDimensions=3  BreakpointsForDimension1=Vcc_Esw_Erec  BreakpointsForDimension2=LossSpec_Diode(m).If_Erec  BreakpointsForDimension3=LossSpec_Diode(m).Tj_Erec  Table=Esw_Erec  RndMeth=Simplest  InputSameDT=on
  Add1 : Sum
  Compare To Zero : simulink/Logic and Bit Operations/Compare To Zero  relop===  OutDataTypeStr=boolean
  Compare To Zero1 : simulink/Logic and Bit Operations/Compare To Zero  relop=>  OutDataTypeStr=boolean
  Energy-to-Power 1 : Subsystem  mask{PulseDuration=PulseDuration, Ts=Ts}
      mask prompts: PulseDuration "Pulse Duration (s):"; Ts "Sample time (s):"
  Logical Operator : Logic  AllPortsSameDT=off  OutDataTypeStr=float('double')
  Memory2 : Memory
  Product : Product  RndMeth=Zero
  Product1 : Product  RndMeth=Zero
  Saturation1 : Saturate  UpperLimit=inf  LowerLimit=0
  Saturation2 : Saturate  UpperLimit=inf  LowerLimit=0
  Selector2 : Selector  InputPortWidth=4  IndexOptions=Index vector (dialog)  Indices="[ 1  3 ]"  OutputSizes=1
  Selector3 : Selector  InputPortWidth=4  IndexOptions=Index vector (dialog)  Indices=[ 2 4 ]  OutputSizes=1
  Psw : Outport
  Pcond : Outport  Port=2
  Ptot : Outport  Port=3
  wires:
  Energy-to-Power 1/1(P_W) -> Saturation2/1
  Product1/1 -> Energy-to-Power 1/2(E_mJ)
  Product/1 -> Saturation1/1
  Tj_C/1 -> 2-D Lookup Table_Vf_on_Diode_Pcond/1, 3-D Lookup Table_Erec_Diode/3
  2-D Lookup Table_Vf_on_Diode_Pcond/1 -> Product/1  "Vf_on_Diode"
  Add1/1 -> Ptot/1
  Compare To Zero1/1 -> Logical Operator/1
  Compare To Zero/1 -> Logical Operator/2
  Logical Operator/1 -> Product1/1, Energy-to-Power 1/1(Trig)
  3-D Lookup Table_Erec_Diode/1 -> Product1/2  "Erec_mJ"
  Selector2/1 -> Memory2/1, Compare To Zero/1, 2-D Lookup Table_Vf_on_Diode_Pcond/2, Product/2  "If"
  mDiode/1 -> Selector2/1, Selector3/1
  Selector3/1 -> 3-D Lookup Table_Erec_Diode/1
  Memory2/1 -> Compare To Zero1/1, 3-D Lookup Table_Erec_Diode/2
  Saturation2/1 -> Psw/1, Add1/1
  Saturation1/1 -> Pcond/1, Add1/2

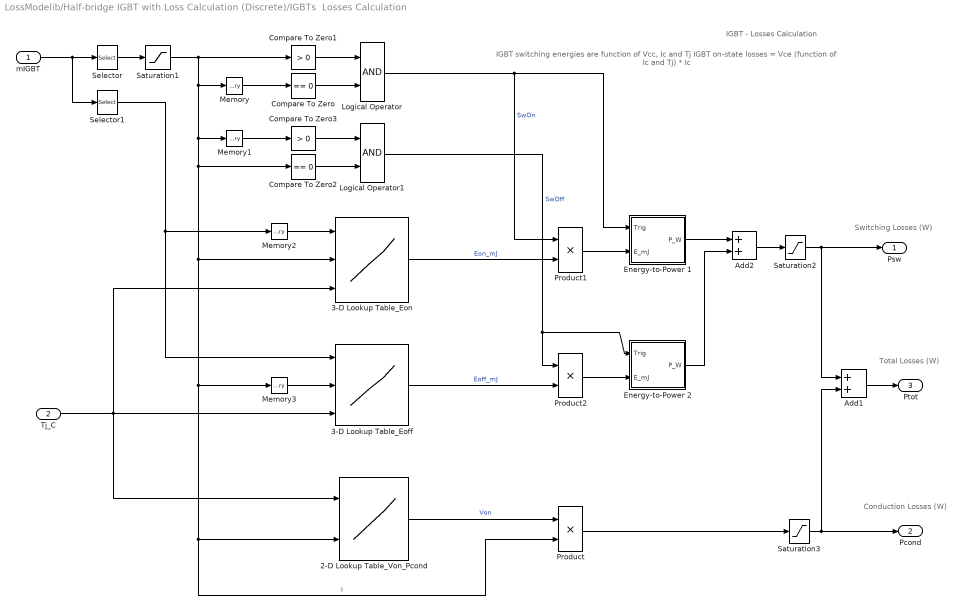
== system LossModelib/Half-bridge IGBT with Loss Calculation (Discrete)/IGBTs  Losses Calculation ==
  note: IGBT switching energies are function of Vcc, Ic and Tj
      | IGBT on-state losses = Vce (function of Ic and Tj) * Ic
  note: Total Losses (W)
  note: Conduction Losses (W)
  note: Switching Losses (W)
  note: IGBT - Losses Calculation
  mIGBT : Inport  PortDimensions=4
  Tj_C : Inport  Port=2
  2-D Lookup Table_Von_Pcond : Lookup_n-D  BreakpointsForDimension1=LossSpec_IGBT(n).Tj_OnState  BreakpointsForDimension2=LossSpec_IGBT(n).Ic_OnState  BreakpointsForDimension3=Page_Temp_C  Table=LossSpec_IGBT(n).Vce_OnState  RndMeth=Simplest  InputSameDT=on
  3-D Lookup Table_Eoff : Lookup_n-D  NumberOfTableDimensions=3  BreakpointsForDimension1=Vcc_Esw_Off  BreakpointsForDimension2=LossSpec_IGBT(n).Ic_Eoff  BreakpointsForDimension3=LossSpec_IGBT(n).Tj_Eoff  Table=Esw_Off  RndMeth=Simplest  InputSameDT=on
  3-D Lookup Table_Eon : Lookup_n-D  NumberOfTableDimensions=3  BreakpointsForDimension1=Vcc_Esw_On  BreakpointsForDimension2=LossSpec_IGBT(n).Ic_Eon  BreakpointsForDimension3=LossSpec_IGBT(n).Tj_Eon  Table=Esw_On  RndMeth=Simplest  InputSameDT=on
  Add1 : Sum
  Add2 : Sum
  Compare To Zero : simulink/Logic and Bit Operations/Compare To Zero  relop===  OutDataTypeStr=boolean
  Compare To Zero1 : simulink/Logic and Bit Operations/Compare To Zero  relop=>  OutDataTypeStr=boolean
  Compare To Zero2 : simulink/Logic and Bit Operations/Compare To Zero  relop===  OutDataTypeStr=boolean
  Compare To Zero3 : simulink/Logic and Bit Operations/Compare To Zero  relop=>  OutDataTypeStr=boolean
  Energy-to-Power 1 : Subsystem  mask{PulseDuration=PulseDuration, Ts=Ts}
      mask prompts: PulseDuration "Pulse Duration (s):"; Ts "Sample time (s):"
  Energy-to-Power 2 : Subsystem  mask{PulseDuration=PulseDuration, Ts=Ts}
      mask prompts: PulseDuration "Pulse Duration (s):"; Ts "Sample time (s):"
  Logical Operator : Logic  AllPortsSameDT=off  OutDataTypeStr=float('double')
  Logical Operator1 : Logic  AllPortsSameDT=off  OutDataTypeStr=float('double')
  Memory{,1..3} (4 alike) : Memory
  Product : Product  RndMeth=Zero
  Product1 : Product  RndMeth=Zero
  Product2 : Product  RndMeth=Zero
  Saturation1 : Saturate  UpperLimit=inf  LowerLimit=0
  Saturation2 : Saturate  UpperLimit=inf  LowerLimit=0
  Saturation3 : Saturate  UpperLimit=inf  LowerLimit=0
  Selector : Selector  InputPortWidth=4  IndexOptions=Index vector (dialog)  Indices="[ 1  3 ]"  OutputSizes=1
  Selector1 : Selector  InputPortWidth=4  IndexOptions=Index vector (dialog)  Indices=[ 2 4 ]  OutputSizes=1
  Psw : Outport
  Pcond : Outport  Port=2
  Ptot : Outport  Port=3
  wires:
  Energy-to-Power 2/1(P_W) -> Add2/2
  Product2/1 -> Energy-to-Power 2/2(E_mJ)
  Product1/1 -> Energy-to-Power 1/2(E_mJ)
  Energy-to-Power 1/1(P_W) -> Add2/1
  2-D Lookup Table_Von_Pcond/1 -> Product/1  "Von"
  Tj_C/1 -> 3-D Lookup Table_Eoff/3, 2-D Lookup Table_Von_Pcond/1, 3-D Lookup Table_Eon/3
  Product/1 -> Saturation3/1
  3-D Lookup Table_Eoff/1 -> Product2/2  "Eoff_mJ"
  3-D Lookup Table_Eon/1 -> Product1/2  "Eon_mJ"
  Memory3/1 -> 3-D Lookup Table_Eoff/2
  Memory2/1 -> 3-D Lookup Table_Eon/1
  Selector/1 -> Saturation1/1
  Add1/1 -> Ptot/1
  mIGBT/1 -> Selector/1, Selector1/1
  Memory/1 -> Compare To Zero/1
  Saturation1/1 -> Compare To Zero1/1, Memory/1, Memory1/1, 3-D Lookup Table_Eon/2, Memory3/1, 2-D Lookup Table_Von_Pcond/2, Product/2, Compare To Zero2/1  "I"
  Compare To Zero1/1 -> Logical Operator/1
  Compare To Zero/1 -> Logical Operator/2
  Logical Operator/1 -> Product1/1, Energy-to-Power 1/1(Trig)  "SwOn"
  Selector1/1 -> Memory2/1, 3-D Lookup Table_Eoff/1
  Compare To Zero3/1 -> Logical Operator1/1
  Compare To Zero2/1 -> Logical Operator1/2
  Logical Operator1/1 -> Product2/1, Energy-to-Power 2/1(Trig)  "SwOff"
  Memory1/1 -> Compare To Zero3/1
  Add2/1 -> Saturation2/1
  Saturation2/1 -> Psw/1, Add1/1
  Saturation3/1 -> Pcond/1, Add1/2

== system LossModelib/Half-bridge IGBT with Loss Calculation (Discrete)/Simscape Interface ==
  Pin : Inport
  Add1 : Sum  Inputs=+-
  Heat Flow Source : fl_lib/Thermal/Thermal Sources/Ideal Heat Flow Source  Q_Log=off  T_Log=off  LocalVarNames=|Q|T  LocalVarDescs=|Q|T  LocalVarLogging=[0 0]
  K1 : Constant  Value=273
  PS-Simulink Converter : nesl_utility/PS-Simulink Converter  PhysicalDomain=network_engine_domain  LeftPortType=input  RightPortType=output  SubClassName=ps_output  Unit=1  AffineConversion=off
  Simulink-PS Converter1 : nesl_utility/Simulink-PS Converter  PhysicalDomain=network_engine_domain  LeftPortType=input  RightPortType=output  SubClassName=ps_input  Unit=1  AffineConversion=off  InputFilterTimeConstant=1e-4  UdotUserProvided=0
  Temperature Sensor : fl_lib/Thermal/Thermal Sensors/Ideal Temperature Sensor  Qs_Log=off  Ts_Log=off  LocalVarNames=|Qs|Ts  LocalVarDescs=|Qs|Ts  LocalVarLogging=[0 0]
  Thermal  Reference1 : fl_lib/Thermal/Thermal Elements/Thermal Reference  Q_Log=off  LocalVarNames=|Q  LocalVarDescs=|Q  LocalVarLogging=0
  Thermal  Reference4 : fl_lib/Thermal/Thermal Elements/Thermal Reference  Q_Log=off  LocalVarNames=|Q  LocalVarDescs=|Q  LocalVarLogging=0
  H : PMIOPort  Port=1  Side=Left
  Tcase : Outport
  wires:
  Pin/1 -> Simulink-PS Converter1/1
  K1/1 -> Add1/2
  PS-Simulink Converter/1 -> Add1/1
  Add1/1 -> Tcase/1
  connections:
  Temperature Sensor/RConn1 -- Thermal  Reference1/LConn1
  Temperature Sensor/RConn2 -- PS-Simulink Converter/LConn1
  Simulink-PS Converter1/RConn1 -- Heat Flow Source/RConn1
  Temperature Sensor/LConn1 -- Heat Flow Source/LConn1 -- H/RConn1
  Thermal  Reference4/LConn1 -- Heat Flow Source/RConn2

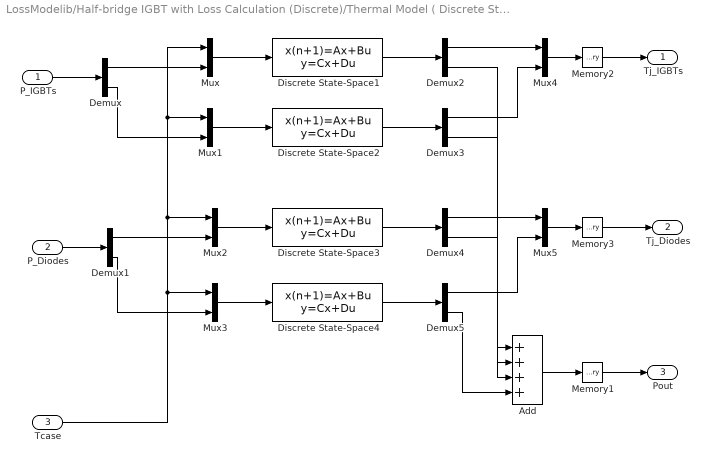
== system LossModelib/Half-bridge IGBT with Loss Calculation (Discrete)/Thermal Model ( Discrete State-Space) ==
  P_IGBTs : Inport  PortDimensions=2
  P_Diodes : Inport  Port=2  PortDimensions=2
  Tcase : Inport  Port=3  PortDimensions=1
  Add : Sum  Inputs=++++
  Demux{,1..5} (6 alike) : Demux  Outputs=2
  Discrete State-Space1 : DiscreteStateSpace  A=Ad_IGBT  B=Bd_IGBT  C=Cd_IGBT  D=Dd_IGBT  X0=x0d  SampleTime=Ts
  Discrete State-Space2 : DiscreteStateSpace  A=Ad_IGBT  B=Bd_IGBT  C=Cd_IGBT  D=Dd_IGBT  X0=x0d  SampleTime=Ts
  Discrete State-Space3 : DiscreteStateSpace  A=Ad_Diode  B=Bd_Diode  C=Cd_Diode  D=Dd_Diode  X0=x0d  SampleTime=Ts
  Discrete State-Space4 : DiscreteStateSpace  A=Ad_Diode  B=Bd_Diode  C=Cd_Diode  D=Dd_Diode  X0=x0d  SampleTime=Ts
  Memory1 : Memory
  Memory2 : Memory  X0=Tj0
  Memory3 : Memory  X0=Tj0
  Mux{,1..5} (6 alike) : Mux  Inputs=2
  Tj_IGBTs : Outport
  Tj_Diodes : Outport  Port=2
  Pout : Outport  Port=3
  wires:
  Memory2/1 -> Tj_IGBTs/1
  Memory3/1 -> Tj_Diodes/1
  Memory1/1 -> Pout/1
  Tcase/1 -> Mux2/1, Mux1/1, Mux/1, Mux3/1
  P_Diodes/1 -> Demux1/1
  P_IGBTs/1 -> Demux/1
  Mux5/1 -> Memory3/1
  Demux5/2 -> Add/4
  Demux4/2 -> Add/3
  Demux3/2 -> Add/2
  Demux2/2 -> Add/1
  Demux5/1 -> Mux5/2
  Demux4/1 -> Mux5/1
  Mux4/1 -> Memory2/1
  Demux3/1 -> Mux4/2
  Demux2/1 -> Mux4/1
  Demux1/2 -> Mux3/2
  Demux/2 -> Mux1/2
  Demux/1 -> Mux/2
  Demux1/1 -> Mux2/2
  Add/1 -> Memory1/1
  Discrete State-Space4/1 -> Demux5/1
  Discrete State-Space3/1 -> Demux4/1
  Discrete State-Space2/1 -> Demux3/1
  Discrete State-Space1/1 -> Demux2/1
  Mux/1 -> Discrete State-Space1/1
  Mux1/1 -> Discrete State-Space2/1
  Mux2/1 -> Discrete State-Space3/1
  Mux3/1 -> Discrete State-Space4/1

== system LossModelib/Half-bridge IGBT with Loss Calculation (Continuous)/Determine currents in IGBTs vs. Diodes/Subsystem1 ==
  I : Inport
  Gain1 : Gain  Gain=-1
  Saturation2 : Saturate  UpperLimit=1e6  LowerLimit=0
  Saturation3 : Saturate  UpperLimit=0  LowerLimit=-1e6
  I_Q : Outport
  I_D : Outport  Port=2
  wires:
  Gain1/1 -> I_D/1
  Saturation2/1 -> I_Q/1
  I/1 -> Saturation3/1, Saturation2/1
  Saturation3/1 -> Gain1/1

== system LossModelib/Half-bridge IGBT with Loss Calculation (Continuous)/Determine currents in IGBTs vs. Diodes/Subsystem2 ==
  I : Inport
  Gain1 : Gain  Gain=-1
  Saturation2 : Saturate  UpperLimit=1e6  LowerLimit=0
  Saturation3 : Saturate  UpperLimit=0  LowerLimit=-1e6
  I_Q : Outport
  I_D : Outport  Port=2
  wires:
  Saturation3/1 -> Gain1/1
  I/1 -> Saturation2/1, Saturation3/1
  Saturation2/1 -> I_Q/1
  Gain1/1 -> I_D/1

== system LossModelib/Half-bridge IGBT with Loss Calculation (Continuous)/Diodes Loss Calculation/Energy-to-Power  ==
  Trig : Inport
  E_mJ : Inport  Port=2
  Constant1 : Constant  Value=1/PulseDuration
  Constant2 : Constant
  Constant3 : Constant  Value=0
  E2P_W : Gain  Gain=1e-3/PulseDuration
  Integrator Limited : Integrator  ExternalReset=rising  InitialCondition=-1  LimitOutput=on  UpperSaturationLimit=0
  Product1 : Product  RndMeth=Zero
  Sample & Hold : powerlib_extras/Control  Blocks/Sample & Hold  ic=0
  Switch1 : Switch  Criteria=u2 ~= 0
  P_W : Outport
  wires:
  Trig/1 -> Integrator Limited/2, Sample & Hold/2
  E_mJ/1 -> E2P_W/1
  E2P_W/1 -> Sample & Hold/1
  Sample & Hold/1 -> Product1/1
  Integrator Limited/1 -> Switch1/2
  Constant1/1 -> Integrator Limited/1
  Constant2/1 -> Switch1/1
  Constant3/1 -> Switch1/3
  Switch1/1 -> Product1/2
  Product1/1 -> P_W/1

== system LossModelib/Half-bridge IGBT with Loss Calculation (Continuous)/IGBTs  Loss Calculation/Energy-to-Power ==
  Trig : Inport
  E_mJ : Inport  Port=2
  Constant1 : Constant  Value=1/PulseDuration
  Constant2 : Constant
  Constant3 : Constant  Value=0
  E2P_W : Gain  Gain=1e-3/PulseDuration
  Integrator Limited : Integrator  ExternalReset=rising  InitialCondition=-1  LimitOutput=on  UpperSaturationLimit=0
  Product1 : Product  RndMeth=Zero
  Sample & Hold : powerlib_extras/Control  Blocks/Sample & Hold  ic=0
  Switch1 : Switch  Criteria=u2 ~= 0
  P_W : Outport
  wires:
  Trig/1 -> Integrator Limited/2, Sample & Hold/2
  E_mJ/1 -> E2P_W/1
  E2P_W/1 -> Sample & Hold/1
  Sample & Hold/1 -> Product1/1
  Integrator Limited/1 -> Switch1/2
  Constant1/1 -> Integrator Limited/1
  Constant2/1 -> Switch1/1
  Constant3/1 -> Switch1/3
  Switch1/1 -> Product1/2
  Product1/1 -> P_W/1

== system LossModelib/Half-bridge IGBT with Loss Calculation (Continuous)/IGBTs  Loss Calculation/Energy-to-Power  ==
  Trig : Inport
  E_mJ : Inport  Port=2
  Constant1 : Constant  Value=1/PulseDuration
  Constant2 : Constant
  Constant3 : Constant  Value=0
  E2P_W : Gain  Gain=1e-3/PulseDuration
  Integrator Limited : Integrator  ExternalReset=rising  InitialCondition=-1  LimitOutput=on  UpperSaturationLimit=0
  Product1 : Product  RndMeth=Zero
  Sample & Hold : powerlib_extras/Control  Blocks/Sample & Hold  ic=0
  Switch1 : Switch  Criteria=u2 ~= 0
  P_W : Outport
  wires:
  Product1/1 -> P_W/1
  Switch1/1 -> Product1/2
  Constant3/1 -> Switch1/3
  Constant2/1 -> Switch1/1
  Constant1/1 -> Integrator Limited/1
  Integrator Limited/1 -> Switch1/2
  Sample & Hold/1 -> Product1/1
  E2P_W/1 -> Sample & Hold/1
  E_mJ/1 -> E2P_W/1
  Trig/1 -> Sample & Hold/2, Integrator Limited/2

== system LossModelib/Half-bridge IGBT with Loss Calculation (Discrete)/Determine currents in IGBTs vs. Diodes/Subsystem1 ==
  I : Inport
  Gain1 : Gain  Gain=-1
  Saturation2 : Saturate  UpperLimit=1e6  LowerLimit=0
  Saturation3 : Saturate  UpperLimit=0  LowerLimit=-1e6
  I_Q : Outport
  I_D : Outport  Port=2
  wires:
  Gain1/1 -> I_D/1
  Saturation2/1 -> I_Q/1
  I/1 -> Saturation3/1, Saturation2/1
  Saturation3/1 -> Gain1/1

== system LossModelib/Half-bridge IGBT with Loss Calculation (Discrete)/Determine currents in IGBTs vs. Diodes/Subsystem2 ==
  I : Inport
  Gain1 : Gain  Gain=-1
  Saturation2 : Saturate  UpperLimit=1e6  LowerLimit=0
  Saturation3 : Saturate  UpperLimit=0  LowerLimit=-1e6
  I_Q : Outport
  I_D : Outport  Port=2
  wires:
  Saturation3/1 -> Gain1/1
  I/1 -> Saturation2/1, Saturation3/1
  Saturation2/1 -> I_Q/1
  Gain1/1 -> I_D/1

== system LossModelib/Half-bridge IGBT with Loss Calculation (Discrete)/Diodes Losses Calculation/Energy-to-Power 1 ==
  Trig : Inport
  E_mJ : Inport  Port=2
  Constant2 : Constant
  Constant3 : Constant  Value=0
  Discrete Monostable : powerlib_extras/Discrete  Control Blocks/Discrete Monostable  EdgeDetect=Rising  t_mono=ceil(PulseDuration/Ts)*Ts  ic=0  Ts=Ts
  Discrete Sample & Hold : powerlib_extras/Discrete  Control Blocks/Discrete Sample & Hold  ic=0  Ts=Ts
  Product1 : Product  RndMeth=Zero
  Switch1 : Switch  Criteria=u2 ~= 0
  gain : Gain  Gain=1e-3/(ceil(PulseDuration/Ts)*Ts)
  P_W : Outport
  wires:
  Product1/1 -> P_W/1
  Discrete Sample & Hold/1 -> Product1/1
  gain/1 -> Discrete Sample & Hold/1
  Trig/1 -> Discrete Sample & Hold/2, Discrete Monostable/1
  E_mJ/1 -> gain/1
  Discrete Monostable/1 -> Switch1/2
  Constant2/1 -> Switch1/1
  Constant3/1 -> Switch1/3
  Switch1/1 -> Product1/2

== system LossModelib/Half-bridge IGBT with Loss Calculation (Discrete)/IGBTs  Losses Calculation/Energy-to-Power 1 ==
  Trig : Inport
  E_mJ : Inport  Port=2
  Constant2 : Constant
  Constant3 : Constant  Value=0
  Discrete Monostable : powerlib_extras/Discrete  Control Blocks/Discrete Monostable  EdgeDetect=Rising  t_mono=ceil(PulseDuration/Ts)*Ts  ic=0  Ts=Ts
  Discrete Sample & Hold : powerlib_extras/Discrete  Control Blocks/Discrete Sample & Hold  ic=0  Ts=Ts
  Product1 : Product  RndMeth=Zero
  Switch1 : Switch  Criteria=u2 ~= 0
  gain : Gain  Gain=1e-3/(ceil(PulseDuration/Ts)*Ts)
  P_W : Outport
  wires:
  Switch1/1 -> Product1/2
  Constant3/1 -> Switch1/3
  Constant2/1 -> Switch1/1
  Discrete Monostable/1 -> Switch1/2
  E_mJ/1 -> gain/1
  Trig/1 -> Discrete Monostable/1, Discrete Sample & Hold/2
  gain/1 -> Discrete Sample & Hold/1
  Discrete Sample & Hold/1 -> Product1/1
  Product1/1 -> P_W/1

== system LossModelib/Half-bridge IGBT with Loss Calculation (Discrete)/IGBTs  Losses Calculation/Energy-to-Power 2 ==
  Trig : Inport
  E_mJ : Inport  Port=2
  Constant2 : Constant
  Constant3 : Constant  Value=0
  Discrete Monostable : powerlib_extras/Discrete  Control Blocks/Discrete Monostable  EdgeDetect=Rising  t_mono=ceil(PulseDuration/Ts)*Ts  ic=0  Ts=Ts
  Discrete Sample & Hold : powerlib_extras/Discrete  Control Blocks/Discrete Sample & Hold  ic=0  Ts=Ts
  Product1 : Product  RndMeth=Zero
  Switch1 : Switch  Criteria=u2 ~= 0
  gain : Gain  Gain=1e-3/(ceil(PulseDuration/Ts)*Ts)
  P_W : Outport
  wires:
  Product1/1 -> P_W/1
  Discrete Sample & Hold/1 -> Product1/1
  gain/1 -> Discrete Sample & Hold/1
  Trig/1 -> Discrete Sample & Hold/2, Discrete Monostable/1
  E_mJ/1 -> gain/1
  Discrete Monostable/1 -> Switch1/2
  Constant2/1 -> Switch1/1
  Constant3/1 -> Switch1/3
  Switch1/1 -> Product1/2
